simulink model "MicroMouseTemplate"  (R2024a)
settings: Solver=FixedStepAuto  StartTime=0.0  StopTime=10.0  RelTol=1e-3  EnableMultiTasking=on
undefined symbols (not defined in the file): samplingTime
libraries: simulink x1
settings Model: STM32="{\"DigitalPortWrite\":[{\"ID\":\"MicroMouseTemplate:84:10\"},{\"ID\":\"MicroMouseTemplate:84:9\"},{\"ID\":\"MicroMouseTemplate:84:8\"},{\"ID\":\"MicroMouseTemplate:84:7\"},{\"ID\":\"MicroMouseTemplate:84:6\"},{\"ID\":\"MicroMouseTemplate:84:5\"},{\"ID\":\"MicroMouseTemplate:84:4\"},{\"ID\":\"MicroMouseTemplate:84:3\"},{\"ID\":\"MicroMouseTemplate:160:19\"},{\"ID\":\"MicroMouseTemplate:2479:4\"},{\"ID\":\"MicroMouseTemplate:2479:6\"},{\"ID\":\"MicroMouseTemplate:2479:7\"},{\"ID\":\"MicroMouseTemplate:2479:8\"},{\"ID\":\"MicroMouseTemplate:2582:3\"},{\"ID\":\"MicroMouseTemplate:2582:4\"},{\"ID\":\"MicroMouseTemplate:2582:5\"},{\"ID\":\"MicroMouseTemplate:2582:2508\"},{\"ID\":\"MicroMouseTemplate:2582:6\"},{\"ID\":\"MicroMouseTemplate:2582:2507\"},{\"ID\":\"MicroMouseTemplate:2582:7\"},{\"ID\":\"MicroMouseTemplate:2582:2538\"},{\"ID\":\"MicroMouseTemplate:2582:8\"},{\"ID\":\"MicroMouseTemplate:2582:2589\"},{\"ID\":\"MicroMouseTemplate:2582:9\"},{\"ID\":\"MicroMouseTemplate:2582:10\"},{\"ID\":\"MicroMouseTemplate:2582:2539\"}],\"PWMOutput\":[{\"ID\":\"MicroMouseTemplate:160:25\"},{\"ID\":\"MicroMouseTemplate:160:24\"}],\"AnalogInput\":{\"ID\":\"MicroMouseTemplate:2357:1\"},\"DigitalPortRead\":[{\"ID\":\"MicroMouseTemplate:2483:3\"},{\"ID\":\"MicroMouseTemplate:2483:4\"}]}"  SimulationMode=external  ExtModeTrigDuration=10  Creator=JesseJabezArendse  LastModifiedBy=masha
settings SolverCC: AllowMultiTaskInputOutput=on  AutoInsertRateTranBlk=on  InsertRTBMode=Never (minimum delay)
settings OptimizationCC: EnhancedBackFolding=on  PassReuseOutputArgsAs=Individual arguments  StateBitsets=on  DataBitsets=on  ZeroExternalMemoryAtStartup=off  ZeroInternalMemoryAtStartup=off  NoFixptDivByZeroProtection=on  MaxStackSize=64  OptimizeBlockOrder=speed  DifferentSizesBufferReuse=on  EfficientTunableParamExpr=on
settings DebuggingCC: MultiTaskCondExecSysMsg=none  ParameterOverflowMsg=none  ParameterPrecisionLossMsg=none  ParameterTunabilityLossMsg=error
settings HardwareCC: ProdBitPerPointer=32  ProdBitPerSizeT=32  ProdBitPerPtrDiffT=32  ProdLargestAtomicInteger=Long  ProdLargestAtomicFloat=Double  ProdWordSize=32  ProdLongLongMode=on  ProdHWDeviceType=ARM Compatible->ARM Cortex  TargetBitPerPointer=64  TargetBitPerSizeT=64  TargetBitPerPtrDiffT=64  TargetLongLongMode=on  TargetIntDivRoundTo=Zero  TargetEndianess=LittleEndian  TargetWordSize=64  TargetHWDeviceType=MATLAB Host
settings ModelReferenceCC: EnableParallelModelReferenceBuilds=on  ParallelModelReferenceMATLABWorkerInit=Copy Base Workspace  SupportModelReferenceSimTargetCustomCode=on
settings SFSimCC: MATLABDynamicMemAlloc=off  SimHardwareAcceleration=native
settings RTWCC: Description=Embedded Coder  SystemTargetFile=ert.tlc  HardwareBoard=STM32L4xx Based  TLCOptions=-p0 -aInlineSetEventsForThisBaseRateFcn=TLC_FALSE -aSuppressMultiTaskScheduler=TLC_FALSE -aRateBasedStepFcn=1  TemplateMakefile=ert_default_tmf  Toolchain=GNU Tools for ARM Embedded Processors  CodeExecutionProfiling=on  CodeProfilingInstrumentation=coarse  GPUComputeCapability=3.5
settings RTWCC: CustomHeaderCode=|
  | #include "MicroMouseProgramming\Core\Inc\IMU.h"
  | #include "MicroMouseProgramming\Core\Inc\CustomWhile.h"
  | #include "MicroMouseProgramming\Core\Inc\Motors.h"
settings RTWCC: CustomInclude=|
  | MicroMouseProgramming\Core\Inc\
  | MicroMouseProgramming\Core\Src\
settings RTWCC: CustomSource=|
  | MicroMouseProgramming\Core\Src\IMU.c
  | MicroMouseProgramming\Core\Src\CustomWhile.c
  | MicroMouseProgramming\Core\Src\Motors.c
settings CodeAppCC: ForceParamTrailComments=on  IgnoreCustomStorageClasses=off  OperatorAnnotations=on  SimulinkDataObjDesc=on  SFDataObjDesc=on  InsertBlockDesc=on
settings ERTTargetCC: CodeReplacementLibrary=ARM Cortex-M  SupportNonFinite=off  SupportComplex=off  ExtModeTransport=3  ExtModeStaticAlloc=on  ExtModeStaticAllocSize=2048  ExtModeMexFile=ext_xcp  ExtModeIntrfLevel=Level2 - Open

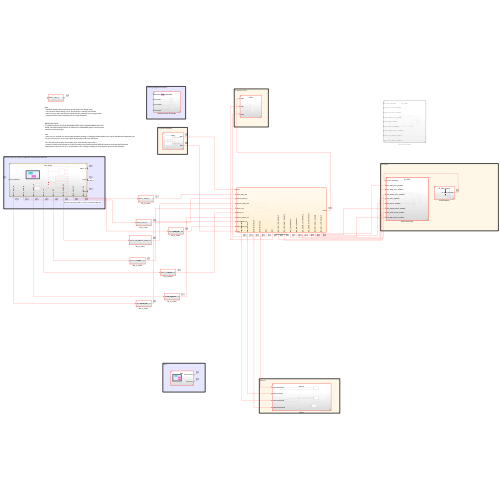
[thumbnail: Simulink's stored preview of the top-level diagram]
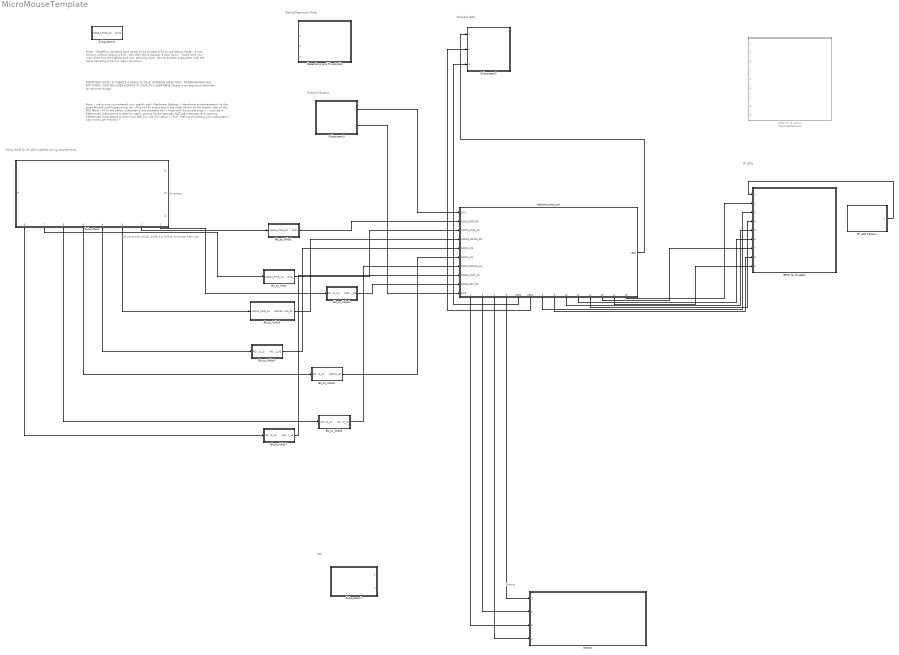
== system MicroMouseTemplate ==
  note: IMPORTANT NOTE:
      | IF THERE'S A SPACE IN YOUR WORKING DIRECTORY, PROGRAMMING WILL NOT WORK, THIS INCLUDES A SPACE IN YOUR PC's USERNAME (Space is an argument delimiter for terminal things)
  note: Note:
      | - make sure you entered your specifc path (Hardware Settings > Hardware Implementation) to the given MicroMouseProgramming.ioc
      | - All given 8x arrays are in the order shown at the bottom side of the ADC Block
      |
      | - fill in the yellow subsystems and probably don't mess with the purple ones :)
      | - working in Referenced Subsystems is ideal for easily porting blocks between MATLAB instances, and opening Referenced Subsystems on their own lets you use Simulation > Run, making simulating your subsystems way more user friendly!!!
  note: 8x arrays
  note: all ports are uint16, 4095 == 3V3 to minimize RAM use
  note: IMU
  note: Fancy Stuff for IR ADCs specific timing requirements
  note: IR LEDs
  note: Motors
  note: Onboard Buttons
  note: Onboard LEDs
  note: Debug/Diagnostic Mode
  note: Note:
      | - Stateflow sampling time needs to be at least 0.05 to use debug mode
      | - a nice amount without debug is 0.01, less than this is actually a slow down
      | - make sure your main chart has the highest and only sampling time, having another
      | subsystem with the same sampling time is a major slowdown
  Bit_to_Volts : Subsystem
  Bit_to_Volts1 : Subsystem
  Bit_to_Volts2 : Subsystem
  Bit_to_Volts3 : Subsystem
  Bit_to_Volts4 : Subsystem
  Bit_to_Volts5 : Subsystem
  Bit_to_Volts6 : Subsystem
  Bit_to_Volts7 : Subsystem
  Detections and Thresholds : Subsystem  ReferencedSubsystem=DiagnosticMode
  GPIO for IR LEDs : Subsystem  TreatAsAtomicUnit=on  SystemSampleTime=samplingTime  ReferencedSubsystem=IR_LEDs
  GPIO for IR LEDs1 : Subsystem  Commented=on  TreatAsAtomicUnit=on  SystemSampleTime=samplingTime  ReferencedSubsystem=IR_LEDs
  HelloMicroMouse! : Stateflow chart  TreatAsAtomicUnit=on
      settings: PortSchema="{\"entries\":[{\"content\":{\"sides\":[{\"content\":{\"connectorIds\":[\"In2\",\"In3\",\"In4\",\"In5\",\"In6\",\"In7\",\"In8\",\"In9\",\"In10\",\"In1\"]},\"type\":\"ConnectorPlacement.EquallySpacedRectSide\",\"uuid\":\"f52daa4f-6374-42e5-9ef1-0ccc99d09b58\"},{\"content\":{\"connectorIds\":[\"Out1\"],\"side\":\"RIGHT\"},\"type\":\"ConnectorPlacement.EquallySpacedRectSide\",\"uuid\":\"94b478cc-4dde-45c7-a588-77cf2b43cdb7\"},{\"content\":{\"side\":\"TOP\"},\"type\":\"ConnectorPlacement.EquallySpacedRectSide\",\"uuid\":\"afff2079-ea5c-423e-9722-09c3bbce433b\"},{\"content\":{\"connectorIds\":[\"Out2\",\"Out3\",\"Out4\",\"Out5\",\"Out6\",\"Out7\",\"Out8\",\"Out9\",\"Out10\",\"Out11\",\"Out12\",\"Out13\",\"Out14\",\"Out15\"],\"side\":\"BOTTOM\"},\"type\":\"ConnectorPlacement.EquallySpacedRectSide\",\"uuid\":\"94e93a1d-795d-41a3-b2d8-d520b2bf47ef\"}]},\"type\":\"ConnectorPlacement.EquallySpacedConnector\",\"uuid\":\"d4d35636-54af-48ac-af70-d56caef5e090\"}],\"packageUris\":[\"http://schema.mathworks.com/mf0/Connector/R2020b\"],\"version\":\"1.0\"}"
  IR LED Pattern : Subsystem  ReferencedSubsystem=IR_LED_Pattern
  Motors : Subsystem  ReferencedSubsystem=Motors
  Subsystem : Subsystem  ReferencedSubsystem=ADC_Block
      settings: PortSchema="{\"entries\":[{\"content\":{\"sides\":[{\"content\":{},\"type\":\"ConnectorPlacement.EquallySpacedRectSide\",\"uuid\":\"be6b81d5-7a49-4e34-b35f-0c07892094fc\"},{\"content\":{\"connectorIds\":[\"Out1\",\"Out2\",\"Out3\",\"Out4\",\"Out5\",\"Out6\",\"Out7\",\"Out8\"],\"side\":\"RIGHT\"},\"type\":\"ConnectorPlacement.EquallySpacedRectSide\",\"uuid\":\"5e22590a-b7c0-4c63-8de4-8d81fd6c3849\"},{\"content\":{\"connectorIds\":[\"Out12\",\"Out10\",\"Out11\"],\"side\":\"TOP\"},\"type\":\"ConnectorPlacement.EquallySpacedRectSide\",\"uuid\":\"da97636e-cea0-4a10-8fe5-d807f9ee999f\"},{\"content\":{\"connectorIds\":[\"Out9\"],\"side\":\"BOTTOM\"},\"type\":\"ConnectorPlacement.EquallySpacedRectSide\",\"uuid\":\"a593d780-81a8-4730-a8bc-2bbf356cafe4\"}]},\"type\":\"ConnectorPlacement.EquallySpacedConnector\",\"uuid\":\"0bcac921-e51a-4437-9183-315712d0a8c2\"}],\"packageUris\":[\"http://schema.mathworks.com/mf0/Connector/R2020b\"],\"version\":\"1.0\"}"
  Subsystem1 : Subsystem  ReferencedSubsystem=IMU
  Subsystem2 : Subsystem  ReferencedSubsystem=LEDs
  Subsystem3 : Subsystem  ReferencedSubsystem=SWs
  Subsystem4 : Subsystem
  wires:
  Subsystem3/1 -> HelloMicroMouse!/2(SW1)
  Subsystem3/2 -> HelloMicroMouse!/1(SW2)
  HelloMicroMouse!/1(LED0) -> Subsystem2/1
  HelloMicroMouse!/2(leftWheelbackward) -> Motors/3
  HelloMicroMouse!/5(rightWheelforward) -> Motors/1
  HelloMicroMouse!/4(rightWheelbackward) -> Motors/4
  HelloMicroMouse!/3(leftWheelforward) -> Motors/2
  HelloMicroMouse!/6(LED2) -> Subsystem2/3
  Bit_to_Volts/1(Out1) -> HelloMicroMouse!/4(ADC14_FWD_LS)
  Subsystem/7 -> Bit_to_Volts/1(ADC14_FWD_LS)
  Bit_to_Volts1/1(Out1) -> HelloMicroMouse!/3(ADC9_FWD_RS)
  Subsystem/2 -> Bit_to_Volts1/1(ADC14_FWD_LS)
  HelloMicroMouse!/7(LED1) -> Subsystem2/2
  IR LED Pattern/1 -> GPIO for IR LEDs/1
  HelloMicroMouse!/8(LED_FWD_LEFT_ENABLE) -> GPIO for IR LEDs/3
  HelloMicroMouse!/9(LED_FWD_RIGHT_ENABLE) -> GPIO for IR LEDs/8
  HelloMicroMouse!/10(LED_LEFT_ENABLE) -> GPIO for IR LEDs/5
  HelloMicroMouse!/11(LED_RIGHT_ENABLE) -> GPIO for IR LEDs/6
  HelloMicroMouse!/15(LED_MOT_LEFT_ENABLE) -> GPIO for IR LEDs/2
  HelloMicroMouse!/12(LED_DOWN_LEFT_ENABLE) -> GPIO for IR LEDs/4
  HelloMicroMouse!/13(LED_DOWN_RIGHT_ENABLE) -> GPIO for IR LEDs/7
  HelloMicroMouse!/14(LED_MOT_RIGHT_ENABLE) -> GPIO for IR LEDs/9
  Subsystem/1 -> Bit_to_Volts2/1(ADC14_FWD_LS)
  Bit_to_Volts2/1(ADC8_MOT_RS) -> HelloMicroMouse!/10(ADC8_MOT_RS)
  Subsystem/3 -> Bit_to_Volts3/1(ADC14_FWD_LS)
  Bit_to_Volts3/1(ADC10_DOWN_RS) -> HelloMicroMouse!/5(ADC10_DOWN_RS)
  Subsystem/4 -> Bit_to_Volts4/1(ADC14_FWD_LS)
  Bit_to_Volts4/1(ADC11_RS) -> HelloMicroMouse!/6(ADC11_RS)
  Subsystem/5 -> Bit_to_Volts5/1(ADC14_FWD_LS)
  Bit_to_Volts5/1(ADC12_LS) -> HelloMicroMouse!/7(ADC12_LS)
  Bit_to_Volts6/1(ADC13_DOWN_LS) -> HelloMicroMouse!/8(ADC13_DOWN_LS)
  Subsystem/6 -> Bit_to_Volts6/1(ADC14_FWD_LS)
  Subsystem/8 -> Bit_to_Volts7/1(ADC14_FWD_LS)
  Bit_to_Volts7/1(ADC15_MOT_LS) -> HelloMicroMouse!/9(ADC15_MOT_LS)

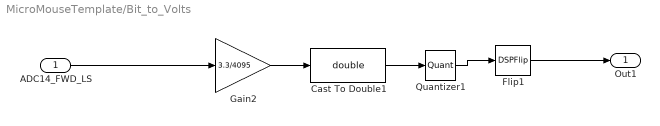
== system MicroMouseTemplate/Bit_to_Volts ==
  ADC14_FWD_LS : Inport
  Cast To Double1 : DataTypeConversion  OutDataTypeStr=double  SaturateOnIntegerOverflow=off  RndMeth=Floor
  Flip1 : DSPFlip
  Gain2 : Gain  Gain=3.3/4095
  Quantizer1 : Quantizer  QuantizationInterval=0.01
  Out1 : Outport
  wires:
  Quantizer1/1 -> Flip1/1
  Gain2/1 -> Cast To Double1/1
  Cast To Double1/1 -> Quantizer1/1
  ADC14_FWD_LS/1 -> Gain2/1
  Flip1/1 -> Out1/1

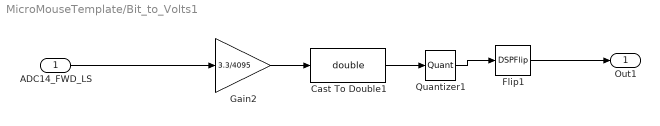
== system MicroMouseTemplate/Bit_to_Volts1 ==
  ADC14_FWD_LS : Inport
  Cast To Double1 : DataTypeConversion  OutDataTypeStr=double  SaturateOnIntegerOverflow=off  RndMeth=Floor
  Flip1 : DSPFlip
  Gain2 : Gain  Gain=3.3/4095
  Quantizer1 : Quantizer  QuantizationInterval=0.01
  Out1 : Outport
  wires:
  Quantizer1/1 -> Flip1/1
  Gain2/1 -> Cast To Double1/1
  Cast To Double1/1 -> Quantizer1/1
  ADC14_FWD_LS/1 -> Gain2/1
  Flip1/1 -> Out1/1

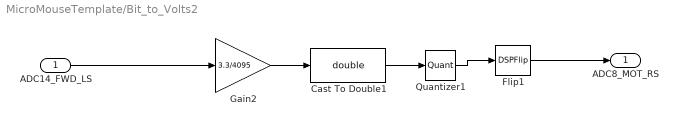
== system MicroMouseTemplate/Bit_to_Volts2 ==
  ADC14_FWD_LS : Inport
  Cast To Double1 : DataTypeConversion  OutDataTypeStr=double  SaturateOnIntegerOverflow=off  RndMeth=Floor
  Flip1 : DSPFlip
  Gain2 : Gain  Gain=3.3/4095
  Quantizer1 : Quantizer  QuantizationInterval=0.01
  ADC8_MOT_RS : Outport
  wires:
  Quantizer1/1 -> Flip1/1
  Gain2/1 -> Cast To Double1/1
  Cast To Double1/1 -> Quantizer1/1
  ADC14_FWD_LS/1 -> Gain2/1
  Flip1/1 -> ADC8_MOT_RS/1

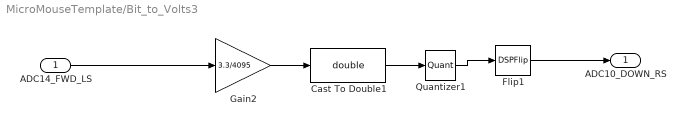
== system MicroMouseTemplate/Bit_to_Volts3 ==
  ADC14_FWD_LS : Inport
  Cast To Double1 : DataTypeConversion  OutDataTypeStr=double  SaturateOnIntegerOverflow=off  RndMeth=Floor
  Flip1 : DSPFlip
  Gain2 : Gain  Gain=3.3/4095
  Quantizer1 : Quantizer  QuantizationInterval=0.01
  ADC10_DOWN_RS : Outport
  wires:
  Quantizer1/1 -> Flip1/1
  Gain2/1 -> Cast To Double1/1
  Cast To Double1/1 -> Quantizer1/1
  ADC14_FWD_LS/1 -> Gain2/1
  Flip1/1 -> ADC10_DOWN_RS/1

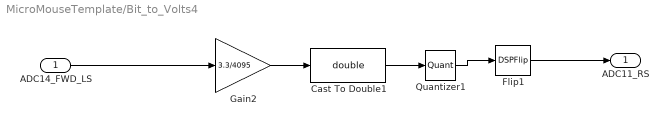
== system MicroMouseTemplate/Bit_to_Volts4 ==
  ADC14_FWD_LS : Inport
  Cast To Double1 : DataTypeConversion  OutDataTypeStr=double  SaturateOnIntegerOverflow=off  RndMeth=Floor
  Flip1 : DSPFlip
  Gain2 : Gain  Gain=3.3/4095
  Quantizer1 : Quantizer  QuantizationInterval=0.01
  ADC11_RS : Outport
  wires:
  Quantizer1/1 -> Flip1/1
  Gain2/1 -> Cast To Double1/1
  Cast To Double1/1 -> Quantizer1/1
  ADC14_FWD_LS/1 -> Gain2/1
  Flip1/1 -> ADC11_RS/1

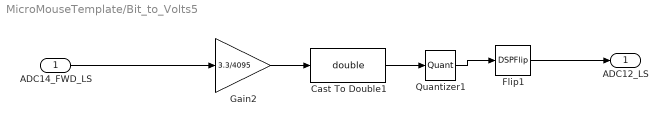
== system MicroMouseTemplate/Bit_to_Volts5 ==
  ADC14_FWD_LS : Inport
  Cast To Double1 : DataTypeConversion  OutDataTypeStr=double  SaturateOnIntegerOverflow=off  RndMeth=Floor
  Flip1 : DSPFlip
  Gain2 : Gain  Gain=3.3/4095
  Quantizer1 : Quantizer  QuantizationInterval=0.01
  ADC12_LS : Outport
  wires:
  Quantizer1/1 -> Flip1/1
  Gain2/1 -> Cast To Double1/1
  Cast To Double1/1 -> Quantizer1/1
  ADC14_FWD_LS/1 -> Gain2/1
  Flip1/1 -> ADC12_LS/1

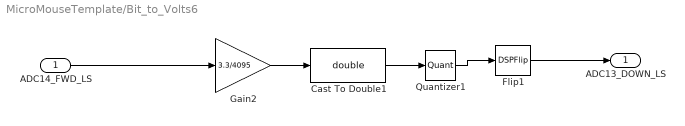
== system MicroMouseTemplate/Bit_to_Volts6 ==
  ADC14_FWD_LS : Inport
  Cast To Double1 : DataTypeConversion  OutDataTypeStr=double  SaturateOnIntegerOverflow=off  RndMeth=Floor
  Flip1 : DSPFlip
  Gain2 : Gain  Gain=3.3/4095
  Quantizer1 : Quantizer  QuantizationInterval=0.01
  ADC13_DOWN_LS : Outport
  wires:
  Quantizer1/1 -> Flip1/1
  Gain2/1 -> Cast To Double1/1
  Cast To Double1/1 -> Quantizer1/1
  ADC14_FWD_LS/1 -> Gain2/1
  Flip1/1 -> ADC13_DOWN_LS/1

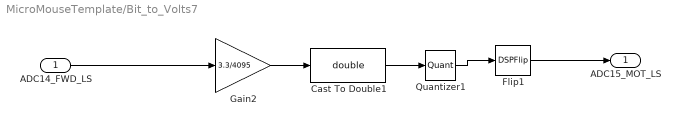
== system MicroMouseTemplate/Bit_to_Volts7 ==
  ADC14_FWD_LS : Inport
  Cast To Double1 : DataTypeConversion  OutDataTypeStr=double  SaturateOnIntegerOverflow=off  RndMeth=Floor
  Flip1 : DSPFlip
  Gain2 : Gain  Gain=3.3/4095
  Quantizer1 : Quantizer  QuantizationInterval=0.01
  ADC15_MOT_LS : Outport
  wires:
  Quantizer1/1 -> Flip1/1
  Gain2/1 -> Cast To Double1/1
  Cast To Double1/1 -> Quantizer1/1
  ADC14_FWD_LS/1 -> Gain2/1
  Flip1/1 -> ADC15_MOT_LS/1

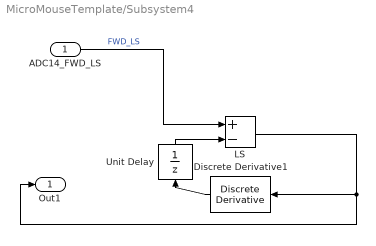
== system MicroMouseTemplate/Subsystem4 ==
  ADC14_FWD_LS : Inport
  Discrete Derivative1 : simulink/Discrete/Discrete Derivative  gainval=0.1  ICPrevScaledInput=0.0  OutMin=[]  OutMax=[]  OutDataTypeStr=uint16  OutputDataTypeScalingMode=uint16  OutDataType=fixdt(1, 16)  OutScaling=2^-10  DoSatur=off
  LS : Sum  Inputs=+-  OutDataTypeStr=uint16  AccumDataTypeStr=uint16
  Unit Delay : UnitDelay  SampleTime=-1  HasFrameUpgradeWarning=on
  Out1 : Outport  OutDataTypeStr=uint16
  wires:
  LS/1 -> Out1/1, Discrete Derivative1/1
  ADC14_FWD_LS/1 -> LS/1  "FWD_LS"
  Discrete Derivative1/1 -> Unit Delay/1
  Unit Delay/1 -> LS/2

== stateflow chart MicroMouseTemplate/HelloMicroMouse! ==
  state ButtonPressed [commented out]
    entry:
    state Right [commented out]
      entry:
      LED0 = false;
      LED1 = true;
      LED2 = false;
      leftWheelforward = 0;
      rightWheelforward = 3000;
      leftWheelbackward = 3000;
      rightWheelbackward = 0;
    state Left [commented out]
      entry:
      LED0 = true;
      LED1 = true;
      LED2 = true;
      leftWheelforward = 3000;
      rightWheelforward = 3000;
      leftWheelbackward = 0;
      rightWheelbackward = 0;
    (default) -> ButtonPressed.Left [commented out]
    ButtonPressed.Left -> ButtonPressed.Right [commented out] : [ADC14_FWD_LS > baseline+.2]
    ButtonPressed.Right -> ButtonPressed.Left [commented out] : after(1,sec)
  state Baseline [commented out]
    entry:
    if (ADC14_FWD_LS < baseline)
    baseline = ADC14_FWD_LS;
    end
    if (baseline < 1.5)
    LED1 = true;
    LED0 = false;
    LED2 = false;
    else
    LED1 = false;
    LED0 = false;
    LED2 = false;
    end
    if (baseline < 2)
    LED2 = true;
    LED0 = false;
    LED1 = false;
    else
    LED2 = false;
    LED1 = false;
    LED0 = false;
    end
  state WaitUntilButtonPressed [commented out]
    during:
    LED0 = true;
    LED1 = false;
    LED2 = false;
    leftWheelforward = 0;
    rightWheelforward = 0;
    leftWheelbackward = 0;
    rightWheelbackward = 0;
    baseline = 3.3;
  state Stop [commented out]
    entry:
    LED0 = false;
    LED1 = false;
    LED2 = false;
    leftWheelforward = 0;
    rightWheelforward = 0;
    leftWheelbackward = 0;
    rightWheelbackward = 0;
  state Baseline4
    during:
    while (counter <= c)
    counter = counter+1;
    sum_LS_FWD = sum_LS_FWD + ADC14_FWD_LS;
    sum_RS_FWD  = ADC9_FWD_RS + sum_RS_FWD;
    sum_MOT_LS = sum_MOT_LS+ADC15_MOT_LS;
    sum_DOWN_LS = ADC13_DOWN_LS+sum_DOWN_LS;
    sum_LS=ADC12_LS+sum_LS;
    sum_RS=sum_RS+ADC11_RS;
    sum_DOWN_RS=sum_DOWN_RS+ADC10_DOWN_RS;
    sum_MOT_RS=sum_MOT_RS+ADC8_MOT_RS;
    end
    baseline_LS_FWD = sum_LS_FWD / counter;
    baseline_RS_FWD = sum_RS_FWD / counter;
    baseline_MOT_LS = sum_MOT_LS/counter;
    baseline_LS = sum_MOT_LS/counter;
    baseline_DOWN_LS = sum_DOWN_LS/counter;
    baseline_RS = sum_RS/counter;
    baseline_DOWN_RS = sum_DOWN_RS/counter;
    baseline_MOT_RS = sum_MOT_RS/counter;
  state Empty_Path1
    entry:
    state LEFT
      during:
      leftWheelforward = 0;
      rightWheelforward = 3000;
      leftWheelbackward = 3000;
      rightWheelbackward = 0;
      LED0=true;
    state FORWARD
      during:
      LED0 = false;
      LED1 = false;
      LED2 = false;
      LED_LEFT_ENABLE=0;
      LED_RIGHT_ENABLE=0;
      LED_FWD_LEFT_ENABLE=1;
      LED_FWD_RIGHT_ENABLE=1;
      leftWheelforward = 3000;
      rightWheelforward = 3000;
      leftWheelbackward = 0;
      rightWheelbackward = 0;
    state SCAN
      during:
      LED_FWD_LEFT_ENABLE=0;
      LED_FWD_RIGHT_ENABLE=0;
      LED_LEFT_ENABLE=1;
      LED_RIGHT_ENABLE=1;
      leftWheelforward = 0;
      rightWheelforward = 0;
      leftWheelbackward = 0;
      rightWheelbackward = 0;
    state RIGHT
      entry:
      leftWheelforward = 3000;
      rightWheelforward = 0;
      leftWheelbackward = 0;
      rightWheelbackward = 3000;
      LED2=true;
    state OneEightyDegreeTurn
      entry:
      leftWheelforward = 3000;
      rightWheelforward = 0;
      leftWheelbackward = 0;
      rightWheelbackward = 3000;
      LED1=true;
    state STOP
      entry:
      leftWheelforward = 0;
      rightWheelforward = 0;
      leftWheelbackward = 0;
      rightWheelbackward = 0;
    Empty_Path1.LEFT -> Empty_Path1.FORWARD : after(1,sec)
    Empty_Path1.SCAN -> Empty_Path1.LEFT [order 1] : [ADC12_LS >baseline_LS+0.5 && ADC11_RS<baseline_RS ]
    (default) -> Empty_Path1.FORWARD
    Empty_Path1.FORWARD -> Empty_Path1.SCAN : [ADC14_FWD_LS > baseline_LS_FWD+.5 || ADC9_FWD_RS > baseline_RS_FWD+.5  ]
    Empty_Path1.SCAN -> Empty_Path1.RIGHT [order 3] : [ADC12_LS > baseline_LS+0.5 && ADC11_RS>baseline_RS+0.5 ]
    Empty_Path1.RIGHT -> Empty_Path1.FORWARD : after(1,sec)
    Empty_Path1.SCAN -> Empty_Path1.OneEightyDegreeTurn [order 2] : [ADC12_LS <baseline_LS && ADC11_RS>baseline_RS+0.5 ]
    Empty_Path1.OneEightyDegreeTurn -> Empty_Path1.STOP : after(2,sec)
  state Baseline_Feedback1
    during:
    if (baseline_LS_FWD || baseline_RS_FWD <= 2)
    LED2 = true;
    end
    if (baseline_LS_FWD || baseline_RS_FWD <= 1.5)
    LED1 = true;
    LED2 = true;
    end
    if (baseline_LS_FWD || baseline_RS_FWD <= 1)
    LED0 = true;
    LED1 = true;
    LED2 = true;
    end
  state Empty_Path [commented out]
    entry:
    state LEFT [commented out]
      during:
      leftWheelforward = 0;
      rightWheelforward = 3000;
      leftWheelbackward = 3000;
      rightWheelbackward = 0;
    state SCAN [commented out]
      during:
      LED_FWD_LEFT_ENABLE=0;
      LED_FWD_RIGHT_ENABLE=0;
      LED_LEFT_ENABLE=1;
      LED_RIGHT_ENABLE=1;
      leftWheelforward = 0;
      rightWheelforward = 3000;
      leftWheelbackward = 3000;
      rightWheelbackward = 0;
    state FORWARD [commented out]
      entry:
      LED_FWD_LEFT_ENABLE=1;
      LED_FWD_RIGHT_ENABLE=1;
      leftWheelforward = 3000;
      rightWheelforward = 3000;
      leftWheelbackward = 0;
      rightWheelbackward = 0;
    state RIGHT [commented out]
      entry:
      leftWheelforward = 3000;
      rightWheelforward = 0;
      leftWheelbackward = 0;
      rightWheelbackward = 3000;
    state OneEightyDegreeTurn [commented out]
      entry:
      leftWheelforward = 3000;
      rightWheelforward = 0;
      leftWheelbackward = 0;
      rightWheelbackward = 3000;
    state STOP [commented out]
      entry:
      leftWheelforward = 0;
      rightWheelforward = 0;
      leftWheelbackward = 0;
      rightWheelbackward = 0;
    Empty_Path.LEFT -> Empty_Path.FORWARD [commented out] : after(1,sec)
    Empty_Path.SCAN -> Empty_Path.LEFT [commented out] : [ADC12_LS >baseline_LS+0.5 && ADC11_RS<baseline_RS ]{LED_LEFT_ENABLE=0;
        | LED_RIGHT_ENABLE=0;}
    (default) -> Empty_Path.FORWARD [commented out]
    Empty_Path.FORWARD -> Empty_Path.SCAN [commented out] : [ADC14_FWD_LS > baseline_LS_FWD+.5 || ADC9_FWD_RS > baseline_RS_FWD+.5  ]
    Empty_Path.SCAN -> Empty_Path.RIGHT [commented out] : [ADC12_LS <baseline_LS && ADC11_RS>baseline_RS+0.5 ]{LED_LEFT_ENABLE=0;
        | LED_RIGHT_ENABLE=0;}
    Empty_Path.OneEightyDegreeTurn -> Empty_Path.FORWARD [commented out] : after(1,sec)
    Empty_Path.SCAN -> Empty_Path.FORWARD [commented out] : after(1.1,sec)
    Empty_Path.SCAN -> Empty_Path.OneEightyDegreeTurn [commented out] : [ADC12_LS > baseline_LS+0.5 && ADC11_RS>baseline_RS+0.5 ]{LED_LEFT_ENABLE=0;
        | LED_RIGHT_ENABLE=0;}
    Empty_Path.OneEightyDegreeTurn -> Empty_Path.STOP [commented out] : after(2,sec)
  state Baseline3 [commented out]
    during:
    while (counter <= c)
    counter = counter+1;
    sum_LS_FWD = sum_LS_FWD + ADC14_FWD_LS;
    sum_RS_FWD  = ADC9_FWD_RS + sum_RS_FWD;
    sum_MOT_LS = sum_MOT_LS+ADC15_MOT_LS;
    sum_DOWN_LS = ADC13_DOWN_LS+sum_DOWN_LS;
    sum_LS=ADC12_LS+sum_LS;
    sum_RS=sum_RS+ADC11_RS;
    sum_DOWN_RS=sum_DOWN_RS+ADC10_DOWN_RS;
    sum_MOT_RS=sum_MOT_RS+ADC8_MOT_RS;
    end
    baseline_LS_FWD = sum_LS_FWD / counter;
    baseline_RS_FWD = sum_RS_FWD / counter;
    baseline_MOT_LS = sum_MOT_LS/counter;
    baseline_LS = sum_MOT_LS/counter;
    baseline_DOWN_LS = sum_DOWN_LS/counter;
    baseline_RS = sum_RS/counter;
    baseline_DOWN_RS = sum_DOWN_RS/counter;
    baseline_MOT_RS = sum_MOT_RS/counter;
    exit:
    LED0 = false;
    LED1 = false;
    LED2 = false;
  state Baseline_Feedback [commented out]
    during:
    if (baseline_LS_FWD || baseline_RS_FWD <= 2)
    LED0 = false;
    LED1 = false;
    LED2 = true;
    end
    if (baseline_LS_FWD || baseline_RS_FWD <= 1.5)
    LED0 = false;
    LED1 = true;
    LED2 = true;
    end
    if (baseline_LS_FWD || baseline_RS_FWD <= 1)
    LED0 = true;
    LED1 = true;
    LED2 = true;
    end
  state Intialization1
    during:
    LED0 = ~LED0;
    LED1 = ~LED1;
    LED2 = ~LED2;
    leftWheelforward = 0;
    rightWheelforward = 0;
    leftWheelbackward = 0;
    rightWheelbackward = 0;
    baseline_LS_FWD =0;
    baseline_RS_FWD=0;
    baseline_MOT_LS=0;
    baseline_DOWN_LS=0;
    baseline_RS=0;
    baseline_LS=0;
    baseline_DOWN_RS=0;
    baseline_MOT_RS=0;
    counter = 0;
    c=50;
    sum_LS_FWD=0;
    sum_RS_FWD=0;
    sum_MOT_LS = 0;
    sum_DOWN_LS = 0;
    sum_LS=0;
    sum_RS=0;
    sum_DOWN_RS=0;
    sum_MOT_RS=0;
    LED_FWD_LEFT_ENABLE=0;
    LED_FWD_RIGHT_ENABLE=0;
    LED_LEFT_ENABLE=0;
    LED_RIGHT_ENABLE=0;
    LED_DOWN_LEFT_ENABLE=0;
    LED_DOWN_RIGHT_ENABLE=0;
    LED_MOT_RIGHT_ENABLE=0;
    LED_MOT_LEFT_ENABLE=0;
  state ButtonPressed1 [commented out]
    entry:
    state Right [commented out]
      entry:
      LED0 = false;
      LED1 = true;
      LED2 = false;
      leftWheelforward = 0;
      rightWheelforward = 3000;
      leftWheelbackward = 3000;
      rightWheelbackward = 0;
    state Left [commented out]
      entry:
      LED0 = true;
      LED1 = true;
      LED2 = true;
      leftWheelforward = 3000;
      rightWheelforward = 3000;
      leftWheelbackward = 0;
      rightWheelbackward = 0;
    (default) -> ButtonPressed1.Left [commented out]
    ButtonPressed1.Left -> ButtonPressed1.Right [commented out] : [ADC14_FWD_LS > baseline+.2]
    ButtonPressed1.Right -> ButtonPressed1.Left [commented out] : after(1,sec)
  state WaitUntilButtonPressed1 [commented out]
    during:
    LED0 = true;
    LED1 = false;
    LED2 = false;
    leftWheelforward = 0;
    rightWheelforward = 0;
    leftWheelbackward = 0;
    rightWheelbackward = 0;
  state Intialization [commented out]
    during:
    LED0 = true;
    LED1 = true;
    LED2 = true;
    leftWheelforward = 0;
    rightWheelforward = 0;
    leftWheelbackward = 0;
    rightWheelbackward = 0;
    baseline_LS_FWD =0;
    baseline_RS_FWD=0;
    baseline_MOT_LS=0;
    baseline_DOWN_LS=0;
    baseline_RS=0;
    baseline_LS=0;
    baseline_DOWN_RS=0;
    baseline_MOT_RS=0;
    counter = 0;
    c=50;
    sum_LS_FWD=0;
    sum_RS_FWD=0;
    sum_MOT_LS = 0;
    sum_DOWN_LS = 0;
    sum_LS=0;
    sum_RS=0;
    sum_DOWN_RS=0;
    sum_MOT_RS=0;
    LED_FWD_LEFT_ENABLE=0;
    LED_FWD_RIGHT_ENABLE=0;
    LED_LEFT_ENABLE=0;
    LED_RIGHT_ENABLE=0;
    LED_DOWN_LEFT_ENABLE=0;
    LED_DOWN_RIGHT_ENABLE=0;
    LED_MOT_RIGHT_ENABLE=0;
    LED_MOT_LEFT_ENABLE=0;
  state Stop4
    entry:
    LED0 = false;
    LED1 = false;
    LED2 = false;
    leftWheelforward = 0;
    rightWheelforward = 0;
    leftWheelbackward = 0;
    rightWheelbackward = 0;
  state Stop1 [commented out]
    entry:
    LED0 = false;
    LED1 = false;
    LED2 = false;
    leftWheelforward = 0;
    rightWheelforward = 0;
    leftWheelbackward = 0;
    rightWheelbackward = 0;
  state Stop3 [commented out]
    entry:
    LED0 = false;
    LED1 = false;
    LED2 = false;
    leftWheelforward = 0;
    rightWheelforward = 0;
    leftWheelbackward = 0;
    rightWheelbackward = 0;
  state ButtonPressed2 [commented out]
    entry:
    state Right [commented out]
      entry:
      leftWheelforward = 0;
      rightWheelforward = 3000;
      leftWheelbackward = 3000;
      rightWheelbackward = 0;
    state Left [commented out]
      entry:
      leftWheelforward = 3000;
      rightWheelforward = 3000;
      leftWheelbackward = 0;
      rightWheelbackward = 0;
    (default) -> ButtonPressed2.Left [commented out]
    ButtonPressed2.Left -> ButtonPressed2.Right [commented out] : [ADC14_FWD_LS > baseline+.5]
    ButtonPressed2.Right -> ButtonPressed2.Left [commented out] : [ADC14_FWD_LS<=baseline]
  state Baseline2 [commented out]
    during:
    if (baseline <= 1)
    LED0 = true;
    LED1 = true;
    LED2 = true;
    end
    if (baseline <= 1.5)
    LED0 = false;
    LED1 = true;
    LED2 = true;
    end
    if (baseline <= 2)
    LED0 = false;
    LED1 = false;
    LED2 = true;
    end
  state Baseline1 [commented out]
    during:
    while (counter <= 50)
    counter = counter+1;
    sum = sum + ADC14_FWD_LS;
    end
    baseline = sum / counter;
    exit:
    LED0 = false;
    LED1 = false;
    LED2 = false;
  state WaitUntilButtonPressed2 [commented out]
    during:
    LED0 = ~LED0;
    LED1 = ~LED1;
    LED2 = ~LED2;
    leftWheelforward = 0;
    rightWheelforward = 0;
    leftWheelbackward = 0;
    rightWheelbackward = 0;
    baseline =0;
    counter = 0;
    sum=0;
  state Stop2 [commented out]
    entry:
    LED0 = false;
    LED1 = false;
    LED2 = false;
    leftWheelforward = 0;
    rightWheelforward = 0;
    leftWheelbackward = 0;
    rightWheelbackward = 0;
  (default) -> WaitUntilButtonPressed [commented out]
  WaitUntilButtonPressed -> Baseline [commented out] : after(5,sec)
  Baseline -> ButtonPressed [commented out] : [SW1==1]
  ButtonPressed -> Stop [commented out] : [SW2==1]
  Stop -> WaitUntilButtonPressed [commented out] : [SW2==1]
  Baseline_Feedback1 -> Empty_Path1 : [SW1==1]
  Baseline4 -> Baseline_Feedback1 : [counter>=c]
  Intialization1 -> Baseline4 : after(2,sec)
  (default) -> Intialization1
  Baseline3 -> Baseline_Feedback [commented out] : [counter>=c]
  Baseline_Feedback -> Empty_Path [commented out] : [SW1==1]
  Intialization -> Baseline3 [commented out] : after(2,sec)
  (default) -> WaitUntilButtonPressed1 [commented out]
  (default) -> Intialization [commented out]
  WaitUntilButtonPressed1 -> ButtonPressed1 [commented out] : [SW1==1]
  Empty_Path1 -> Stop4 : [SW2==1]
  Stop4 -> Intialization1 : [SW2==1]
  ButtonPressed1 -> Stop1 [commented out] : [SW2==1]
  Stop1 -> WaitUntilButtonPressed1 [commented out] : [SW2==1]
  Empty_Path -> Stop3 [commented out] : [SW2==1]
  Stop3 -> Intialization [commented out] : [SW2==1]
  (default) -> WaitUntilButtonPressed2 [commented out]
  Baseline2 -> ButtonPressed2 [commented out] : [SW1==1]
  Baseline1 -> Baseline2 [commented out] : [counter>=50]
  WaitUntilButtonPressed2 -> Baseline1 [commented out] : after(2,sec)
  ButtonPressed2 -> Stop2 [commented out] : [SW2==1]
  Stop2 -> WaitUntilButtonPressed2 [commented out] : [SW2==1]
  data: SW2 input; LED0 output; SW1 input; leftWheelbackward output; leftWheelforward output; rightWheelbackward output; rightWheelforward output; LED2 output; ADC9_FWD_RS input double; ADC14_FWD_LS input double; baseline local; counter local; sum local; baseline_LS_FWD local; baseline_RS_FWD local; sum_LS_FWD local; sum_RS_FWD local; LED1 output; LED_FWD_LEFT_ENABLE output; LED_FWD_RIGHT_ENABLE output; LED_LEFT_ENABLE output; LED_RIGHT_ENABLE output; LED_DOWN_LEFT_ENABLE output; LED_DOWN_RIGHT_ENABLE output; LED_MOT_RIGHT_ENABLE output; LED_MOT_LEFT_ENABLE output; baseline_DOWN_LS local; baseline_DOWN_RS local; baseline_MOT_LS local; baseline_MOT_RS local; baseline_LS local; baseline_RS local; c local; sum_DOWN_LS local; sum_DOWN_RS local; sum_LS local; sum_MOT_LS local; sum_MOT_RS local; sum_RS local; ADC10_DOWN_RS input; ADC11_RS input; ADC12_LS input; ADC13_DOWN_LS input; ADC15_MOT_LS input; ADC8_MOT_RS input
